simulink library "AyazOctLiftingBdy_cl"  (R2018b)
settings: Solver=VariableStepAuto  StartTime=0.0  StopTime=10.0  RelTol=1e-3
undefined symbols (not defined in the file or in its folder): sim_param
settings Model: Creator=asiddiq2  LastModifiedBy=asiddiq2

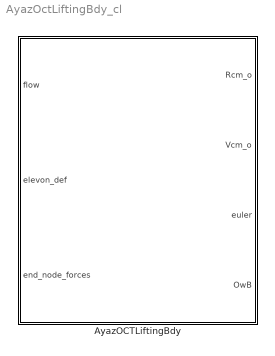
== system AyazOctLiftingBdy_cl ==
  AyazOCTLiftingBdy : Subsystem  mask{sim_param=sim_param, initCon=0}
      mask prompts: sim_param "Simulation parameters structure"; initCon "Initial conditions"

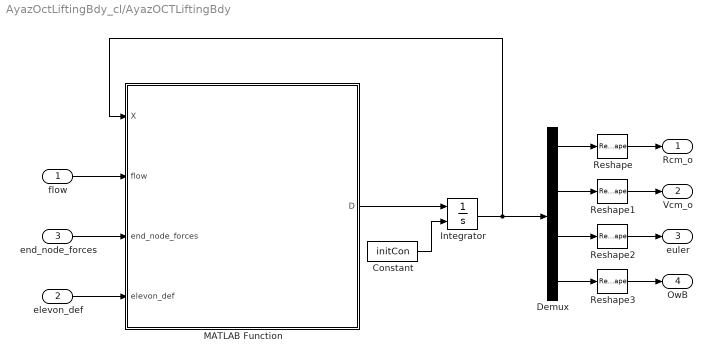
== system AyazOctLiftingBdy_cl/AyazOCTLiftingBdy ==
  flow : Inport
  elevon_def : Inport  Port=2
  end_node_forces : Inport  Port=3
  Constant : Constant  Value=initCon
  Demux : Demux
  Integrator : Integrator  InitialConditionSource=external
  MATLAB Function : MATLAB Function  TreatAsAtomicUnit=on
  Reshape{,1..3} (4 alike) : Reshape  OutputDimensionality=Column vector (2-D)
  Rcm_o : Outport
  Vcm_o : Outport  Port=2
  euler : Outport  Port=3
  OwB : Outport  Port=4
  wires:
  MATLAB Function/1(D) -> Integrator/1
  Integrator/1 -> MATLAB Function/1(X), Demux/1
  Demux/1 -> Reshape/1
  Demux/4 -> Reshape3/1
  Demux/3 -> Reshape2/1
  Demux/2 -> Reshape1/1
  Reshape/1 -> Rcm_o/1
  Reshape1/1 -> Vcm_o/1
  Reshape2/1 -> euler/1
  Reshape3/1 -> OwB/1
  flow/1 -> MATLAB Function/2(flow)
  elevon_def/1 -> MATLAB Function/4(elevon_def)
  end_node_forces/1 -> MATLAB Function/3(end_node_forces)
  Constant/1 -> Integrator/2

== matlab function AyazOctLiftingBdy_cl/AyazOCTLiftingBdy/MATLAB Function ==
  data: X input; D output; flow input; end_node_forces input; elevon_def input; sim_param parameter
function D = multimode_ode(X,flow,end_node_forces,elevon_def,sim_param)

D = zeros(size(X));

% loader = load('sim_param.mat');
% 
% sim_param = loader.sim_param;

% extract other values
mass = sim_param.geom_param.mass;
MI = sim_param.geom_param.MI;

%% constants
m = mass;
Ixx = MI(1,1);
Iyy = MI(2,2);
Izz = MI(3,3);

m_added = sim_param.geom_param.m_added;
Izz_added = sim_param.geom_param.Izz_added;

%% extract values from state space
% lifting body values
Rcm_o = X(1:3,1);
O_Vcm_o = X(4:6,1);

euler_ang = X(7:9,1);
ph = euler_ang(1);
th = euler_ang(2);
ps = euler_ang(3);

% rotations
[oCb,bCo] = rotation_sequence(euler_ang);

OwB = X(10:12,1);
wx = OwB(1);
wy = OwB(2);
wz = OwB(3);


%%  center of mass first derivatives
D(1:3,1) = O_Vcm_o;
D(7,1) = wx + sin(ph)*tan(th)*wy + cos(ph)*tan(th)*wz;
D(8,1) = cos(ph)*wy - sin(ph)*wz;
D(9,1) = sec(th)*sin(ph)*wy + cos(ph)*sec(th)*wz;


%% EXTERNAL FORCES AND TORQUES
op = multinode_F_and_T_external2(sim_param,flow,elevon_def,Rcm_o,...
    O_Vcm_o,OwB,euler_ang,end_node_forces);

O_F_ext = op.O_F_ext;
B_T_ext = op.B_T_ext;

Tx = B_T_ext(1);
Ty = B_T_ext(2);
Tz = B_T_ext(3);

%% center of mass second derivatives
% added mass
mass_matrix = [1/(m+m_added(1)) 0 0;0 1/(m+m_added(2)) 0;0 0 1/(m+m_added(3))];

D(4:6,1) = oCb*(mass_matrix*(bCo*O_F_ext));
D(10,1) = (1/Ixx)*(Tx + (Iyy - Izz)*wy*wz);
D(11,1) = (1/Iyy)*(Ty + (Izz - Ixx)*wx*wz);
D(12,1) = (1/(Izz+Izz_added))*(Tz + (Ixx - Iyy)*wx*wy);


end
